simulink library "lib_fuel_converter3"  (Simulink 10.1)
settings: Solver=VariableStepAuto  StartTime=0.0  StopTime=10.0  RelTol=1e-3
undefined symbols (not defined in the file or in its folder): air_cp, amb_tmp, cyc_mph, ex_gas_cp, fc_acc_mass, fc_base_mass, fc_c2i_th_cond, fc_c_init_tmp, fc_cl2h_eff, fc_CO2_to_FUELgps, fc_cold, fc_cold_tmp, fc_cp, fc_ct_trq, fc_emisv, fc_ext_sarea, fc_fuel_den, fc_fuel_lhv, fc_h2x_th_cond, fc_h_air_flow, fc_h_cp, fc_h_init_tmp, fc_hood_emisv, fc_hood_sarea, fc_i2x_th_cond, fc_i_init_tmp, fc_inertia, fc_map_spd, fc_map_trq, fc_max_trq, fc_pwr_scale, fc_spd_scale, fc_trq_scale, fc_tstat, fc_x_init_tmp, fd_ratio, gb_num_init, gb_ratio, pow, vc_idle_bool, vc_idle_spd, vc_key_on, veh_glider_mass, wh_radius
undefined symbols (not defined in the file): fc_co_map, fc_co_map_c2h, fc_exflow_map, fc_extmp_map, fc_fuel_map, fc_fuel_map_c2h, fc_hc_map, fc_hc_map_c2h, fc_nn_model_name, fc_nox_map, fc_nox_map_c2h, fc_o2_map, fc_pm_map, fc_pm_map_c2h, generalName, logFlag
libraries: $bdroot x4, lib_etc x4, lib_fuel_converter x2, lib_fuel_converter2 x1
(part 2 of 8)

== system lib_fuel_converter3/configurable subsystems/fuel use and EO emis/Block NOTES ==
  note: This block determines actual fuel use and engine-out emissions
      | given the fully hot values and the engine coolant temperature.
      | The correlations used here were developed at NREL using
      | FTP data collected under subcontract by JDM & Associates.
      | Note: PM hot/cold relation assumed same as HC

== system lib_fuel_converter3/configurable subsystems/fuel use and EO emis/HOT engine maps ==
  T (Nm) : Inport
  w (rad/s) : Inport  Port=2
  Enable : EnablePort  StatesWhenEnabling=reset
  Block NOTES : Subsystem
      mask Display: disp('Block\nNOTES')
  CO (g/s) : Subsystem  mask(2-D Table Lookup){xindex=fc_map_spd*fc_spd_scale, yindex=fc_map_trq*fc_trq_scale, table=fc_co_map*fc_spd_scale*fc_trq_scale}
      mask prompts: xindex "X Index"; yindex "Y Index"
      mask help:
      | Two Dimensional Table Lookup
      | The first input corresponds to X Index and the second input corresponds to the Y Index
      mask init:
      | sftab2chk(xindex,yindex,table);
      mask Help: This block returns a linearly interpolated intersection from the table using the X index (which corresponds to the rows of the table) and the Y index (which corresponds to the columns of the table).  Extrapolation is used.
      mask Display: plot(-10,-10,110,110,[90,50,10],[90,40,30],[90,50,10],[50,26,20],[90,50,10],[22,13,10])
  Fcn3 : Fcn  Expr=(u(1)/1000)*ex_gas_cp*(u(2) - amb_tmp)
  HC (g/s) : Subsystem  mask(2-D Table Lookup){xindex=fc_map_spd*fc_spd_scale, yindex=fc_map_trq*fc_trq_scale, table=fc_hc_map*fc_spd_scale*fc_trq_scale}
      mask prompts: xindex "X Index"; yindex "Y Index"
      mask help:
      | Two Dimensional Table Lookup
      | The first input corresponds to X Index and the second input corresponds to the Y Index
      mask init:
      | sftab2chk(xindex,yindex,table);
      mask Help: This block returns a linearly interpolated intersection from the table using the X index (which corresponds to the rows of the table) and the Y index (which corresponds to the columns of the table).  Extrapolation is used.
      mask Display: plot(-10,-10,110,110,[90,50,10],[90,40,30],[90,50,10],[50,26,20],[90,50,10],[22,13,10])
  MF,ex (g/s) : Subsystem  mask(2-D Table Lookup){xindex=fc_map_spd*fc_spd_scale, yindex=fc_map_trq*fc_trq_scale, table=fc_exflow_map*fc_spd_scale*fc_trq_scale}
      mask prompts: xindex "X Index"; yindex "Y Index"
      mask help:
      | Two Dimensional Table Lookup
      | The first input corresponds to X Index and the second input corresponds to the Y Index
      mask init:
      | sftab2chk(xindex,yindex,table);
      mask Help: This block returns a linearly interpolated intersection from the table using the X index (which corresponds to the rows of the table) and the Y index (which corresponds to the columns of the table).  Extrapolation is used.
      mask Display: plot(-10,-10,110,110,[90,50,10],[90,40,30],[90,50,10],[50,26,20],[90,50,10],[22,13,10])
  MinMax : MinMax  Inputs=2
  Mux : Mux
  Mux4 : Mux  Inputs=2
  NOx (g/s) : Subsystem  mask(2-D Table Lookup){xindex=fc_map_spd*fc_spd_scale, yindex=fc_map_trq*fc_trq_scale, table=fc_nox_map*fc_spd_scale*fc_trq_scale}
      mask prompts: xindex "X Index"; yindex "Y Index"
      mask help:
      | Two Dimensional Table Lookup
      | The first input corresponds to X Index and the second input corresponds to the Y Index
      mask init:
      | sftab2chk(xindex,yindex,table);
      mask Help: This block returns a linearly interpolated intersection from the table using the X index (which corresponds to the rows of the table) and the Y index (which corresponds to the columns of the table).  Extrapolation is used.
      mask Display: plot(-10,-10,110,110,[90,50,10],[90,40,30],[90,50,10],[50,26,20],[90,50,10],[22,13,10])
  O2 (g/s) : Subsystem  mask(2-D Table Lookup){xindex=fc_map_spd*fc_spd_scale, yindex=fc_map_trq*fc_trq_scale, table=fc_o2_map*fc_spd_scale*fc_trq_scale}
      mask prompts: xindex "X Index"; yindex "Y Index"
      mask help:
      | Two Dimensional Table Lookup
      | The first input corresponds to X Index and the second input corresponds to the Y Index
      mask init:
      | sftab2chk(xindex,yindex,table);
      mask Help: This block returns a linearly interpolated intersection from the table using the X index (which corresponds to the rows of the table) and the Y index (which corresponds to the columns of the table).  Extrapolation is used.
      mask Display: plot(-10,-10,110,110,[90,50,10],[90,40,30],[90,50,10],[50,26,20],[90,50,10],[22,13,10])
  PM (g/s) : Subsystem  mask(2-D Table Lookup){xindex=fc_map_spd*fc_spd_scale, yindex=fc_map_trq*fc_trq_scale, table=fc_pm_map*fc_spd_scale*fc_trq_scale}
      mask prompts: xindex "X Index"; yindex "Y Index"
      mask help:
      | Two Dimensional Table Lookup
      | The first input corresponds to X Index and the second input corresponds to the Y Index
      mask init:
      | sftab2chk(xindex,yindex,table);
      mask Help: This block returns a linearly interpolated intersection from the table using the X index (which corresponds to the rows of the table) and the Y index (which corresponds to the columns of the table).  Extrapolation is used.
      mask Display: plot(-10,-10,110,110,[90,50,10],[90,40,30],[90,50,10],[50,26,20],[90,50,10],[22,13,10])
  Product : Product  SaturateOnIntegerOverflow=on
  Saturation : Saturate  UpperLimit=max(fc_map_trq*fc_trq_scale)  LowerLimit=min(fc_map_trq*fc_trq_scale)
  Saturation1 : Saturate  UpperLimit=max(fc_map_spd*fc_spd_scale)  LowerLimit=min(fc_map_spd*fc_spd_scale)
  Sum5 : Sum  Inputs=-+  SaturateOnIntegerOverflow=on
  Sum6 : Sum  Inputs=-+  SaturateOnIntegerOverflow=on
  Tex,eo (C) : Subsystem  mask(2-D Table Lookup){xindex=fc_map_spd*fc_spd_scale, yindex=fc_map_trq*fc_trq_scale, table=fc_extmp_map}
      mask prompts: xindex "X Index"; yindex "Y Index"
      mask help:
      | Two Dimensional Table Lookup
      | The first input corresponds to X Index and the second input corresponds to the Y Index
      mask init:
      | sftab2chk(xindex,yindex,table);
      mask Help: This block returns a linearly interpolated intersection from the table using the X index (which corresponds to the rows of the table) and the Y index (which corresponds to the columns of the table).  Extrapolation is used.
      mask Display: plot(-10,-10,110,110,[90,50,10],[90,40,30],[90,50,10],[50,26,20],[90,50,10],[22,13,10])
  fuel (g/s) : Subsystem  mask(2-D Table Lookup){xindex=fc_map_spd*fc_spd_scale, yindex=fc_map_trq*fc_trq_scale, table=fc_fuel_map*fc_spd_scale*fc_trq_scale}
      mask prompts: xindex "X Index"; yindex "Y Index"
      mask help:
      | Two Dimensional Table Lookup
      | The first input corresponds to X Index and the second input corresponds to the Y Index
      mask init:
      | sftab2chk(xindex,yindex,table);
      mask Help: This block returns a linearly interpolated intersection from the table using the X index (which corresponds to the rows of the table) and the Y index (which corresponds to the columns of the table).  Extrapolation is used.
      mask Display: plot(-10,-10,110,110,[90,50,10],[90,40,30],[90,50,10],[50,26,20],[90,50,10],[22,13,10])
  lhv : Gain  Gain=fc_fuel_lhv  SaturateOnIntegerOverflow=on
  fc heat (W) : Outport  OutputWhenDisabled=reset  InitialOutput=eps
  HOT fuel use (g/s) : Outport  Port=2  OutputWhenDisabled=reset  InitialOutput=eps
  HOT emis (g/s) : Outport  Port=3  OutputWhenDisabled=reset  InitialOutput=eps
  Ex Gas Flow (g/s) : Outport  Port=4  OutputWhenDisabled=reset  InitialOutput=eps
  Ex Gas Temp (C) : Outport  Port=5  OutputWhenDisabled=reset  InitialOutput=amb_tmp
  O2 exhaust (g/s) : Outport  Port=6  OutputWhenDisabled=reset  InitialOutput=0
  ex heat (W) : Outport  Port=7  OutputWhenDisabled=reset  InitialOutput=eps
  wires:
  PM (g/s)/1(table out) -> Mux/4
  HC (g/s)/1(table out) -> Mux/1
  CO (g/s)/1(table out) -> Mux/2
  NOx (g/s)/1(table out) -> Mux/3
  Mux/1 -> HOT emis (g/s)/1
  MF,ex (g/s)/1(table out) -> Ex Gas Flow (g/s)/1, Mux4/1
  Tex,eo (C)/1(table out) -> Ex Gas Temp (C)/1, Mux4/2
  Saturation1/1 -> NOx (g/s)/1(x0), MF,ex (g/s)/1(x0), Tex,eo (C)/1(x0), fuel (g/s)/1(x0), O2 (g/s)/1(x0), PM (g/s)/1(x0), CO (g/s)/1(x0), HC (g/s)/1(x0)
  Saturation/1 -> CO (g/s)/2(y0), MF,ex (g/s)/2(y0), Tex,eo (C)/2(y0), fuel (g/s)/2(y0), O2 (g/s)/2(y0), PM (g/s)/2(y0), NOx (g/s)/2(y0), HC (g/s)/2(y0)
  T (Nm)/1 -> Saturation/1, Product/1
  w (rad/s)/1 -> Saturation1/1, Product/2
  Mux4/1 -> Fcn3/1
  Sum5/1 -> fc heat (W)/1
  Fcn3/1 -> MinMax/1
  MinMax/1 -> Sum5/1, ex heat (W)/1
  Sum6/1 -> Sum5/2, MinMax/2
  Product/1 -> Sum6/1
  fuel (g/s)/1(table out) -> HOT fuel use (g/s)/1, lhv/1
  lhv/1 -> Sum6/2
  O2 (g/s)/1(table out) -> O2 exhaust (g/s)/1

== system lib_fuel_converter3/configurable subsystems/fuel use and EO emis/enhancedToWorkspace1 ==
  In1 : Inport
  Terminator : Terminator
  wires:
  In1/1 -> Terminator/1

== system lib_fuel_converter3/configurable subsystems/fuel use and EO emis/enhancedToWorkspace10 ==
  In1 : Inport
  Terminator : Terminator
  wires:
  In1/1 -> Terminator/1

== system lib_fuel_converter3/configurable subsystems/fuel use and EO emis/enhancedToWorkspace11 ==
  In1 : Inport
  Terminator : Terminator
  wires:
  In1/1 -> Terminator/1

== system lib_fuel_converter3/configurable subsystems/fuel use and EO emis/enhancedToWorkspace12 ==
  In1 : Inport
  Terminator : Terminator
  wires:
  In1/1 -> Terminator/1

== system lib_fuel_converter3/configurable subsystems/fuel use and EO emis/enhancedToWorkspace2 ==
  In1 : Inport
  Terminator : Terminator
  wires:
  In1/1 -> Terminator/1

== system lib_fuel_converter3/configurable subsystems/fuel use and EO emis/enhancedToWorkspace3 ==
  In1 : Inport
  Terminator : Terminator
  wires:
  In1/1 -> Terminator/1

== system lib_fuel_converter3/configurable subsystems/fuel use and EO emis/enhancedToWorkspace5 ==
  In1 : Inport
  Terminator : Terminator
  wires:
  In1/1 -> Terminator/1

== system lib_fuel_converter3/configurable subsystems/fuel use and EO emis/enhancedToWorkspace6 ==
  In1 : Inport
  Terminator : Terminator
  wires:
  In1/1 -> Terminator/1

== system lib_fuel_converter3/configurable subsystems/fuel use and EO emis/enhancedToWorkspace7 ==
  In1 : Inport
  Terminator : Terminator
  wires:
  In1/1 -> Terminator/1

== system lib_fuel_converter3/configurable subsystems/fuel use and EO emis/enhancedToWorkspace8 ==
  In1 : Inport
  Terminator : Terminator
  wires:
  In1/1 -> Terminator/1

== system lib_fuel_converter3/configurable subsystems/fuel use and EO emis/enhancedToWorkspace9 ==
  In1 : Inport
  Terminator : Terminator
  wires:
  In1/1 -> Terminator/1

== system lib_fuel_converter3/configurable subsystems/fuel use and EO emis/fc temp ==
  note: h
  note: x
  note: i
  note: c
  veh spd (m/s) : Inport
  key ON? : Inport  Port=2
  fc ON? : Inport  Port=3
  Qfc (W) : Inport  Port=4
  "1/ " : Gain  Gain=1/(0.2*fc_base_mass*fc_pwr_scale*fc_cp)  SaturateOnIntegerOverflow=on
  1/Ci : Gain  Gain=1/(0.8*fc_base_mass*fc_pwr_scale*fc_cp)  SaturateOnIntegerOverflow=on
  1/Cx : Gain  Gain=1/(fc_acc_mass*fc_pwr_scale*fc_cp)  SaturateOnIntegerOverflow=on
  1/mcp : Gain  Gain=1/(0.1*veh_glider_mass*fc_pwr_scale*fc_h_cp)  SaturateOnIntegerOverflow=on
  Block NOTES : Subsystem
      mask Display: disp('Block\nNOTES')
  Memory : Memory  InitialCondition=fc_h_init_tmp
  Mux3 : Mux
  Mux4 : Mux  Inputs=2
  Qc : Sum  SaturateOnIntegerOverflow=on
  Qc1 : Sum  Inputs=--+  SaturateOnIntegerOverflow=on
  Tcm : Integrator  InitialCondition=fc_c_init_tmp
  Tcx : Integrator  InitialCondition=fc_x_init_tmp
  Tcx1 : Integrator  InitialCondition=fc_i_init_tmp
  Tm : Integrator  InitialCondition=fc_h_init_tmp
  fc coolant : Subsystem  TreatAsAtomicUnit=on
  fc mass heat flow : Subsystem
  old fc coolant  temp. (C) : Subsystem
  Tfc_old  (C) : Outport  InitialOutput=0
  Qfc r,h : Outport  Port=2  InitialOutput=0
  Tfc  (C) : Outport  Port=3  InitialOutput=0
  tag scope: fc_hood_temp=scoped
  wires:
  Qc/1 -> "1/ "/1
  "1/ "/1 -> Tcm/1
  Qfc (W)/1 -> Qc/1
  fc mass heat flow/1(Qfc_c) -> Qc/2
  Qc1/1 -> 1/Ci/1
  1/Ci/1 -> Tcx1/1
  Tcm/1 -> Mux3/1
  fc mass heat flow/2(Qfc_i) -> Qc1/3, fc coolant/2("Qfc_i ")
  fc coolant/2(Qfc_htr) -> Qc1/2, Mux4/2
  fc coolant/1(Qfc_rad) -> Qc1/1, Mux4/1
  Tcx1/1 -> fc coolant/1(Tcl), Mux3/2
  Mux4/1 -> Qfc r,h/1
  1/Cx/1 -> Tcx/1
  fc mass heat flow/3(Qfc_x) -> 1/Cx/1
  key ON?/1 -> fc coolant/Enable
  Tcx/1 -> Mux3/3
  Tm/1 -> Mux3/4, Memory/1
  1/mcp/1 -> Tm/1
  fc mass heat flow/4(Qfc_h) -> 1/mcp/1
  Mux3/1 -> fc mass heat flow/2(fc_temp), Tfc  (C)/1
  old fc coolant  temp. (C)/1(fc coolant  temp (C)) -> Tfc_old  (C)/1
  veh spd (m/s)/1 -> old fc coolant  temp. (C)/2(veh spd), fc mass heat flow/1(veh spd)
  fc ON?/1 -> old fc coolant  temp. (C)/1(fc on?)
  Memory/1 -> [fc_hood_temp]

== system lib_fuel_converter3/configurable subsystems/fuel use and EO emis/fc temp correct ==
  Coolant T (C) : Inport
  HOT fuel use (g/s) : Inport  Port=2
  HOT emis (g/s) : Inport  Port=3
  T (Nm) : Inport  Port=4
  w (rad/s) : Inport  Port=5
  Enable : EnablePort  StatesWhenEnabling=reset
  =1: use map based =0: use constant equation based : Constant  Value=fc_cold
  Switch : Switch  Threshold=eps  SaturateOnIntegerOverflow=on  InputSameDT=on
  Switch1 : Switch  Threshold=eps  SaturateOnIntegerOverflow=on  InputSameDT=on
  fc temp correct Constant Correction Factors (Equation Based) : Subsystem  TreatAsAtomicUnit=on
  fc temp correct Variable Correction Factors (Map Based) : Subsystem  TreatAsAtomicUnit=on
  fc_cold=0 : Logic  Operator=NOT
  fuel use (g/s) : Outport  OutputWhenDisabled=reset  InitialOutput=0
  EO emis (g/s) : Outport  Port=2  OutputWhenDisabled=reset  InitialOutput=0
  wires:
  =1: use map based =0: use constant equation based/1 -> fc_cold=0/1, fc temp correct Variable Correction Factors (Map Based)/Enable
  Coolant T (C)/1 -> fc temp correct Constant Correction Factors (Equation Based)/1(Coolant T (C)), fc temp correct Variable Correction Factors (Map Based)/1(Coolant T (C))
  HOT fuel use (g/s)/1 -> fc temp correct Constant Correction Factors (Equation Based)/2(HOT fuel use (g/s)), fc temp correct Variable Correction Factors (Map Based)/2(HOT fuel use (g/s))
  HOT emis (g/s)/1 -> fc temp correct Constant Correction Factors (Equation Based)/3(HOT emis (g/s)), fc temp correct Variable Correction Factors (Map Based)/3(HOT emis (g/s))
  fc temp correct Constant Correction Factors (Equation Based)/1(fuel use (g/s)) -> Switch/1
  fc_cold=0/1 -> fc temp correct Constant Correction Factors (Equation Based)/Enable, Switch/2, Switch1/2
  fc temp correct Variable Correction Factors (Map Based)/1(fuel use (g/s)) -> Switch/3
  fc temp correct Constant Correction Factors (Equation Based)/2(EO emis (g/s)) -> Switch1/1
  fc temp correct Variable Correction Factors (Map Based)/2(EO emis (g/s)) -> Switch1/3
  Switch/1 -> fuel use (g/s)/1
  Switch1/1 -> EO emis (g/s)/1
  T (Nm)/1 -> fc temp correct Variable Correction Factors (Map Based)/4(T (Nm))
  w (rad/s)/1 -> fc temp correct Variable Correction Factors (Map Based)/5(w (rad/s))

== system lib_fuel_converter3/configurable subsystems/fuel use and EO emis Neural Network Model/HOT engine maps ==
  T (Nm) : Inport
  w (rad/s) : Inport  Port=2
  Enable : EnablePort  StatesWhenEnabling=reset
  Block NOTES : Subsystem
      mask Display: disp('Block\nNOTES')
  CO (g/s) : Subsystem  mask(2-D Table Lookup){xindex=fc_map_spd*fc_spd_scale, yindex=fc_map_trq*fc_trq_scale, table=fc_co_map*fc_spd_scale*fc_trq_scale}
      mask prompts: xindex "X Index"; yindex "Y Index"
      mask help:
      | Two Dimensional Table Lookup
      | The first input corresponds to X Index and the second input corresponds to the Y Index
      mask init:
      | sftab2chk(xindex,yindex,table);
      mask Help: This block returns a linearly interpolated intersection from the table using the X index (which corresponds to the rows of the table) and the Y index (which corresponds to the columns of the table).  Extrapolation is used.
      mask Display: plot(-10,-10,110,110,[90,50,10],[90,40,30],[90,50,10],[50,26,20],[90,50,10],[22,13,10])
  Fcn3 : Fcn  Expr=(u(1)/1000)*ex_gas_cp*(u(2) - amb_tmp)
  HC (g/s) : Subsystem  mask(2-D Table Lookup){xindex=fc_map_spd*fc_spd_scale, yindex=fc_map_trq*fc_trq_scale, table=fc_hc_map*fc_spd_scale*fc_trq_scale}
      mask prompts: xindex "X Index"; yindex "Y Index"
      mask help:
      | Two Dimensional Table Lookup
      | The first input corresponds to X Index and the second input corresponds to the Y Index
      mask init:
      | sftab2chk(xindex,yindex,table);
      mask Help: This block returns a linearly interpolated intersection from the table using the X index (which corresponds to the rows of the table) and the Y index (which corresponds to the columns of the table).  Extrapolation is used.
      mask Display: plot(-10,-10,110,110,[90,50,10],[90,40,30],[90,50,10],[50,26,20],[90,50,10],[22,13,10])
  MF,ex (g/s) : Subsystem  mask(2-D Table Lookup){xindex=fc_map_spd*fc_spd_scale, yindex=fc_map_trq*fc_trq_scale, table=fc_exflow_map*fc_spd_scale*fc_trq_scale}
      mask prompts: xindex "X Index"; yindex "Y Index"
      mask help:
      | Two Dimensional Table Lookup
      | The first input corresponds to X Index and the second input corresponds to the Y Index
      mask init:
      | sftab2chk(xindex,yindex,table);
      mask Help: This block returns a linearly interpolated intersection from the table using the X index (which corresponds to the rows of the table) and the Y index (which corresponds to the columns of the table).  Extrapolation is used.
      mask Display: plot(-10,-10,110,110,[90,50,10],[90,40,30],[90,50,10],[50,26,20],[90,50,10],[22,13,10])
  MinMax : MinMax  Inputs=2
  Mux : Mux
  Mux4 : Mux  Inputs=2
  NOx (g/s) : Subsystem  mask(2-D Table Lookup){xindex=fc_map_spd*fc_spd_scale, yindex=fc_map_trq*fc_trq_scale, table=fc_nox_map*fc_spd_scale*fc_trq_scale}
      mask prompts: xindex "X Index"; yindex "Y Index"
      mask help:
      | Two Dimensional Table Lookup
      | The first input corresponds to X Index and the second input corresponds to the Y Index
      mask init:
      | sftab2chk(xindex,yindex,table);
      mask Help: This block returns a linearly interpolated intersection from the table using the X index (which corresponds to the rows of the table) and the Y index (which corresponds to the columns of the table).  Extrapolation is used.
      mask Display: plot(-10,-10,110,110,[90,50,10],[90,40,30],[90,50,10],[50,26,20],[90,50,10],[22,13,10])
  O2 (g/s) : Subsystem  mask(2-D Table Lookup){xindex=fc_map_spd*fc_spd_scale, yindex=fc_map_trq*fc_trq_scale, table=fc_o2_map*fc_spd_scale*fc_trq_scale}
      mask prompts: xindex "X Index"; yindex "Y Index"
      mask help:
      | Two Dimensional Table Lookup
      | The first input corresponds to X Index and the second input corresponds to the Y Index
      mask init:
      | sftab2chk(xindex,yindex,table);
      mask Help: This block returns a linearly interpolated intersection from the table using the X index (which corresponds to the rows of the table) and the Y index (which corresponds to the columns of the table).  Extrapolation is used.
      mask Display: plot(-10,-10,110,110,[90,50,10],[90,40,30],[90,50,10],[50,26,20],[90,50,10],[22,13,10])
  PM (g/s) : Subsystem  mask(2-D Table Lookup){xindex=fc_map_spd*fc_spd_scale, yindex=fc_map_trq*fc_trq_scale, table=fc_pm_map*fc_spd_scale*fc_trq_scale}
      mask prompts: xindex "X Index"; yindex "Y Index"
      mask help:
      | Two Dimensional Table Lookup
      | The first input corresponds to X Index and the second input corresponds to the Y Index
      mask init:
      | sftab2chk(xindex,yindex,table);
      mask Help: This block returns a linearly interpolated intersection from the table using the X index (which corresponds to the rows of the table) and the Y index (which corresponds to the columns of the table).  Extrapolation is used.
      mask Display: plot(-10,-10,110,110,[90,50,10],[90,40,30],[90,50,10],[50,26,20],[90,50,10],[22,13,10])
  Product : Product  SaturateOnIntegerOverflow=on
  Saturation : Saturate  UpperLimit=max(fc_map_trq*fc_trq_scale)  LowerLimit=min(fc_map_trq*fc_trq_scale)
  Saturation1 : Saturate  UpperLimit=max(fc_map_spd*fc_spd_scale)  LowerLimit=min(fc_map_spd*fc_spd_scale)
  Sum5 : Sum  Inputs=-+  SaturateOnIntegerOverflow=on
  Sum6 : Sum  Inputs=-+  SaturateOnIntegerOverflow=on
  Tex,eo (C) : Subsystem  mask(2-D Table Lookup){xindex=fc_map_spd*fc_spd_scale, yindex=fc_map_trq*fc_trq_scale, table=fc_extmp_map}
      mask prompts: xindex "X Index"; yindex "Y Index"
      mask help:
      | Two Dimensional Table Lookup
      | The first input corresponds to X Index and the second input corresponds to the Y Index
      mask init:
      | sftab2chk(xindex,yindex,table);
      mask Help: This block returns a linearly interpolated intersection from the table using the X index (which corresponds to the rows of the table) and the Y index (which corresponds to the columns of the table).  Extrapolation is used.
      mask Display: plot(-10,-10,110,110,[90,50,10],[90,40,30],[90,50,10],[50,26,20],[90,50,10],[22,13,10])
  fuel (g/s) : Subsystem  mask(2-D Table Lookup){xindex=fc_map_spd*fc_spd_scale, yindex=fc_map_trq*fc_trq_scale, table=fc_fuel_map*fc_spd_scale*fc_trq_scale}
      mask prompts: xindex "X Index"; yindex "Y Index"
      mask help:
      | Two Dimensional Table Lookup
      | The first input corresponds to X Index and the second input corresponds to the Y Index
      mask init:
      | sftab2chk(xindex,yindex,table);
      mask Help: This block returns a linearly interpolated intersection from the table using the X index (which corresponds to the rows of the table) and the Y index (which corresponds to the columns of the table).  Extrapolation is used.
      mask Display: plot(-10,-10,110,110,[90,50,10],[90,40,30],[90,50,10],[50,26,20],[90,50,10],[22,13,10])
  lhv : Gain  Gain=fc_fuel_lhv  SaturateOnIntegerOverflow=on
  fc heat (W) : Outport  OutputWhenDisabled=reset  InitialOutput=eps
  HOT fuel use (g/s) : Outport  Port=2  OutputWhenDisabled=reset  InitialOutput=eps
  HOT emis (g/s) : Outport  Port=3  OutputWhenDisabled=reset  InitialOutput=eps
  Ex Gas Flow (g/s) : Outport  Port=4  OutputWhenDisabled=reset  InitialOutput=eps
  Ex Gas Temp (C) : Outport  Port=5  OutputWhenDisabled=reset  InitialOutput=amb_tmp
  O2 exhaust (g/s) : Outport  Port=6  OutputWhenDisabled=reset  InitialOutput=0
  ex heat (W) : Outport  Port=7  OutputWhenDisabled=reset  InitialOutput=eps
  wires:
  PM (g/s)/1(table out) -> Mux/4
  HC (g/s)/1(table out) -> Mux/1
  CO (g/s)/1(table out) -> Mux/2
  NOx (g/s)/1(table out) -> Mux/3
  Mux/1 -> HOT emis (g/s)/1
  MF,ex (g/s)/1(table out) -> Ex Gas Flow (g/s)/1, Mux4/1
  Tex,eo (C)/1(table out) -> Ex Gas Temp (C)/1, Mux4/2
  Saturation1/1 -> NOx (g/s)/1(x0), MF,ex (g/s)/1(x0), Tex,eo (C)/1(x0), fuel (g/s)/1(x0), O2 (g/s)/1(x0), PM (g/s)/1(x0), CO (g/s)/1(x0), HC (g/s)/1(x0)
  Saturation/1 -> CO (g/s)/2(y0), MF,ex (g/s)/2(y0), Tex,eo (C)/2(y0), fuel (g/s)/2(y0), O2 (g/s)/2(y0), PM (g/s)/2(y0), NOx (g/s)/2(y0), HC (g/s)/2(y0)
  T (Nm)/1 -> Saturation/1, Product/1
  w (rad/s)/1 -> Saturation1/1, Product/2
  Mux4/1 -> Fcn3/1
  Sum5/1 -> fc heat (W)/1
  Fcn3/1 -> MinMax/1
  MinMax/1 -> Sum5/1, ex heat (W)/1
  Sum6/1 -> Sum5/2, MinMax/2
  Product/1 -> Sum6/1
  fuel (g/s)/1(table out) -> HOT fuel use (g/s)/1, lhv/1
  lhv/1 -> Sum6/2
  O2 (g/s)/1(table out) -> O2 exhaust (g/s)/1

== system lib_fuel_converter3/configurable subsystems/fuel use and EO emis Neural Network Model/enhancedToWorkspace1 ==
  In1 : Inport
  Terminator : Terminator
  wires:
  In1/1 -> Terminator/1

== system lib_fuel_converter3/configurable subsystems/fuel use and EO emis Neural Network Model/enhancedToWorkspace12 ==
  In1 : Inport
  Terminator : Terminator
  wires:
  In1/1 -> Terminator/1

== system lib_fuel_converter3/configurable subsystems/fuel use and EO emis Neural Network Model/enhancedToWorkspace13 ==
  In1 : Inport
  Terminator : Terminator
  wires:
  In1/1 -> Terminator/1

== system lib_fuel_converter3/configurable subsystems/fuel use and EO emis Neural Network Model/enhancedToWorkspace14 ==
  In1 : Inport
  Terminator : Terminator
  wires:
  In1/1 -> Terminator/1

== system lib_fuel_converter3/configurable subsystems/fuel use and EO emis Neural Network Model/enhancedToWorkspace15 ==
  In1 : Inport
  Terminator : Terminator
  wires:
  In1/1 -> Terminator/1

== system lib_fuel_converter3/configurable subsystems/fuel use and EO emis Neural Network Model/enhancedToWorkspace16 ==
  In1 : Inport
  Terminator : Terminator
  wires:
  In1/1 -> Terminator/1

== system lib_fuel_converter3/configurable subsystems/fuel use and EO emis Neural Network Model/enhancedToWorkspace17 ==
  In1 : Inport
  Terminator : Terminator
  wires:
  In1/1 -> Terminator/1

== system lib_fuel_converter3/configurable subsystems/fuel use and EO emis Neural Network Model/enhancedToWorkspace18 ==
  In1 : Inport
  Terminator : Terminator
  wires:
  In1/1 -> Terminator/1

== system lib_fuel_converter3/configurable subsystems/fuel use and EO emis Neural Network Model/enhancedToWorkspace2 ==
  In1 : Inport
  Terminator : Terminator
  wires:
  In1/1 -> Terminator/1

== system lib_fuel_converter3/configurable subsystems/fuel use and EO emis Neural Network Model/enhancedToWorkspace3 ==
  In1 : Inport
  Terminator : Terminator
  wires:
  In1/1 -> Terminator/1

== system lib_fuel_converter3/configurable subsystems/fuel use and EO emis Neural Network Model/enhancedToWorkspace5 ==
  In1 : Inport
  Terminator : Terminator
  wires:
  In1/1 -> Terminator/1

== system lib_fuel_converter3/configurable subsystems/fuel use and EO emis Neural Network Model/enhancedToWorkspace6 ==
  In1 : Inport
  Terminator : Terminator
  wires:
  In1/1 -> Terminator/1

== system lib_fuel_converter3/configurable subsystems/fuel use and EO emis Neural Network Model/enhancedToWorkspace7 ==
  In1 : Inport
  Terminator : Terminator
  wires:
  In1/1 -> Terminator/1

== system lib_fuel_converter3/configurable subsystems/fuel use and EO emis Neural Network Model/enhancedToWorkspace8 ==
  In1 : Inport
  Terminator : Terminator
  wires:
  In1/1 -> Terminator/1

== system lib_fuel_converter3/configurable subsystems/fuel use and EO emis Neural Network Model/enhancedToWorkspace9 ==
  In1 : Inport
  Terminator : Terminator
  wires:
  In1/1 -> Terminator/1

== system lib_fuel_converter3/configurable subsystems/fuel use and EO emis Neural Network Model/fc temp ==
  note: c
  note: i
  note: x
  note: h
  veh spd (m/s) : Inport
  key ON? : Inport  Port=2
  fc ON? : Inport  Port=3
  Qfc (W) : Inport  Port=4
  "1/ " : Gain  Gain=1/(0.2*fc_base_mass*fc_pwr_scale*fc_cp)  SaturateOnIntegerOverflow=on
  1/Ci : Gain  Gain=1/(0.8*fc_base_mass*fc_pwr_scale*fc_cp)  SaturateOnIntegerOverflow=on
  1/Cx : Gain  Gain=1/(fc_acc_mass*fc_pwr_scale*fc_cp)  SaturateOnIntegerOverflow=on
  1/mcp : Gain  Gain=1/(0.1*veh_glider_mass*fc_pwr_scale*fc_h_cp)  SaturateOnIntegerOverflow=on
  Block NOTES : Subsystem
      mask Display: disp('Block\nNOTES')
  Memory : Memory  InitialCondition=fc_h_init_tmp
  Mux3 : Mux
  Mux4 : Mux  Inputs=2
  Qc : Sum  SaturateOnIntegerOverflow=on
  Qc1 : Sum  Inputs=--+  SaturateOnIntegerOverflow=on
  Tcm : Integrator  InitialCondition=fc_c_init_tmp
  Tcx : Integrator  InitialCondition=fc_x_init_tmp
  Tcx1 : Integrator  InitialCondition=fc_i_init_tmp
  Tm : Integrator  InitialCondition=fc_h_init_tmp
  fc coolant : lib_fuel_converter2/configurable subsystems/fuel use and EO emis Neural Network Model/fc temp/fc coolant  TreatAsAtomicUnit=on
      settings: RTWFcnNameOpts=Auto  RTWFileNameOpts=Auto
  fc mass heat flow : Subsystem
  old fc coolant  temp. (C) : Subsystem
  Tfc_old  (C) : Outport  InitialOutput=0
  Qfc r,h : Outport  Port=2  InitialOutput=0
  Tfc  (C) : Outport  Port=3  InitialOutput=0
  tag scope: fc_hood_temp=scoped
  wires:
  fc ON?/1 -> old fc coolant  temp. (C)/1(fc on?)
  veh spd (m/s)/1 -> fc mass heat flow/1(veh spd), old fc coolant  temp. (C)/2(veh spd)
  old fc coolant  temp. (C)/1(fc coolant  temp (C)) -> Tfc_old  (C)/1
  Mux3/1 -> Tfc  (C)/1, fc mass heat flow/2(fc_temp)
  fc mass heat flow/4(Qfc_h) -> 1/mcp/1
  1/mcp/1 -> Tm/1
  Tm/1 -> Mux3/4, Memory/1
  Tcx/1 -> Mux3/3
  key ON?/1 -> fc coolant/Enable
  fc mass heat flow/3(Qfc_x) -> 1/Cx/1
  1/Cx/1 -> Tcx/1
  Mux4/1 -> Qfc r,h/1
  Tcx1/1 -> Mux3/2, fc coolant/1
  fc coolant/1 -> Mux4/1, Qc1/1
  fc coolant/2 -> Mux4/2, Qc1/2
  fc mass heat flow/2(Qfc_i) -> fc coolant/2, Qc1/3
  Tcm/1 -> Mux3/1
  1/Ci/1 -> Tcx1/1
  Qc1/1 -> 1/Ci/1
  fc mass heat flow/1(Qfc_c) -> Qc/2
  Qfc (W)/1 -> Qc/1
  "1/ "/1 -> Tcm/1
  Qc/1 -> "1/ "/1
  Memory/1 -> [fc_hood_temp]

== system lib_fuel_converter3/configurable subsystems/fuel use and EO emis Neural Network Model/fc temp correct ==
  Coolant T (C) : Inport
  HOT fuel use (g/s) : Inport  Port=2
  HOT emis (g/s) : Inport  Port=3
  T (Nm) : Inport  Port=4
  w (rad/s) : Inport  Port=5
  Enable : EnablePort  StatesWhenEnabling=reset
  =1: use map based =0: use constant equation based : Constant  Value=fc_cold
  Switch : Switch  Threshold=eps  SaturateOnIntegerOverflow=on  InputSameDT=on
  Switch1 : Switch  Threshold=eps  SaturateOnIntegerOverflow=on  InputSameDT=on
  fc temp correct Constant Correction Factors (Equation Based) : Subsystem  TreatAsAtomicUnit=on
  fc temp correct Variable Correction Factors (Map Based) : Subsystem  TreatAsAtomicUnit=on
  fc_cold=0 : Logic  Operator=NOT
  fuel use (g/s) : Outport  OutputWhenDisabled=reset  InitialOutput=0
  EO emis (g/s) : Outport  Port=2  OutputWhenDisabled=reset  InitialOutput=0
  wires:
  w (rad/s)/1 -> fc temp correct Variable Correction Factors (Map Based)/5(w (rad/s))
  T (Nm)/1 -> fc temp correct Variable Correction Factors (Map Based)/4(T (Nm))
  Switch1/1 -> EO emis (g/s)/1
  Switch/1 -> fuel use (g/s)/1
  fc temp correct Variable Correction Factors (Map Based)/2(EO emis (g/s)) -> Switch1/3
  fc temp correct Constant Correction Factors (Equation Based)/2(EO emis (g/s)) -> Switch1/1
  fc temp correct Variable Correction Factors (Map Based)/1(fuel use (g/s)) -> Switch/3
  fc_cold=0/1 -> Switch1/2, Switch/2, fc temp correct Constant Correction Factors (Equation Based)/Enable
  fc temp correct Constant Correction Factors (Equation Based)/1(fuel use (g/s)) -> Switch/1
  HOT emis (g/s)/1 -> fc temp correct Variable Correction Factors (Map Based)/3(HOT emis (g/s)), fc temp correct Constant Correction Factors (Equation Based)/3(HOT emis (g/s))
  HOT fuel use (g/s)/1 -> fc temp correct Variable Correction Factors (Map Based)/2(HOT fuel use (g/s)), fc temp correct Constant Correction Factors (Equation Based)/2(HOT fuel use (g/s))
  Coolant T (C)/1 -> fc temp correct Variable Correction Factors (Map Based)/1(Coolant T (C)), fc temp correct Constant Correction Factors (Equation Based)/1(Coolant T (C))
  =1: use map based =0: use constant equation based/1 -> fc temp correct Variable Correction Factors (Map Based)/Enable, fc_cold=0/1

== system lib_fuel_converter3/configurable subsystems/fuel use and EO emis Neural Network Model/nn thermal calcs ==
  gpsCO2 : Inport
  pwr (W) : Inport  Port=2
  ex gas flow (g/s) : Inport  Port=3
  ex gas tmp : Inport  Port=4
  (g/s CO2) to (g/s fuel) : Gain  Gain=fc_CO2_to_FUELgps  SaturateOnIntegerOverflow=on
  Fcn3 : Fcn  Expr=(u(1)/1000)*ex_gas_cp*(u(2) - amb_tmp)
  MinMax : MinMax  Inputs=2
  Mux4 : Mux  Inputs=2
  Sum5 : Sum  Inputs=-+  SaturateOnIntegerOverflow=on
  Sum6 : Sum  Inputs=-+  SaturateOnIntegerOverflow=on
  lhv : Gain  Gain=fc_fuel_lhv  SaturateOnIntegerOverflow=on
  fc heat (W) : Outport  OutputWhenDisabled=reset  InitialOutput=eps
  HOT fuel use (g/s) : Outport  Port=2  OutputWhenDisabled=reset  InitialOutput=eps
  ex heat (W) : Outport  Port=3  OutputWhenDisabled=reset  InitialOutput=eps
  wires:
  lhv/1 -> Sum6/2
  [fuel_gps] -> lhv/1, HOT fuel use (g/s)/1
  Sum6/1 -> MinMax/2, Sum5/2
  MinMax/1 -> ex heat (W)/1, Sum5/1
  Fcn3/1 -> MinMax/1
  Sum5/1 -> fc heat (W)/1
  Mux4/1 -> Fcn3/1
  gpsCO2/1 -> (g/s CO2) to (g/s fuel)/1
  (g/s CO2) to (g/s fuel)/1 -> [fuel_gps]
  pwr (W)/1 -> Sum6/1
  ex gas tmp/1 -> Mux4/2
  ex gas flow (g/s)/1 -> Mux4/1
